simulink model "cic_dezim4_"  (Simulink 7.8)
settings: Solver=FixedStepDiscrete  StartTime=0.0  StopTime=1  RelTol=1e-3
undefined symbols (not defined in the file or in its folder): dfilt
libraries: dspsigops x8, dspsrcs4 x1, dsparch4 x1
settings Model: Creator=svenhoffmann  LastModifiedBy=josef  ExtModeAutoUpdateStatusClock=off
settings OptimizationCC: InlineInvariantSignals=on  InitFltsAndDblsToZero=on
settings DebuggingCC: SaveWithParameterizedLinksMsg=none  SignalResolutionControl=TryResolveAllWithWarning  MultiTaskDSMMsg=warning  MultiTaskCondExecSysMsg=none  FcnCallInpInsideContextMsg=Use local settings  StrictBusMsg=None
settings RTWCC: IncludeERTFirstTime=on
settings GRTTargetCC: TargetFcnLib=ansi_tfl_tmw.mat

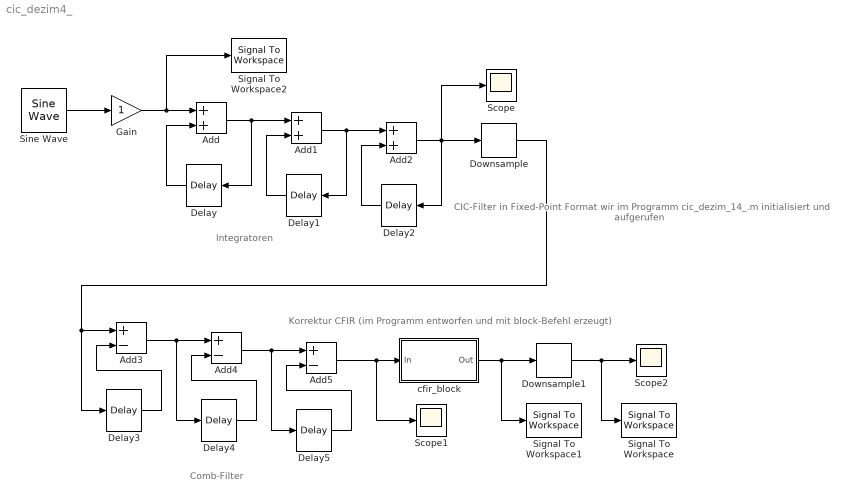
== system cic_dezim4_ ==
  note: Korrektur CFIR (im Programm entworfen
      | und mit block-Befehl erzeugt)
  note: CIC-Filter
      | in Fixed-Point
      | Format
      | wir im Programm
      | cic_dezim_14_.m
      | initialisiert
      | und aufgerufen
  note: Integratoren
  note: Comb-Filter
  Add : Sum  OutDataTypeStr=Inherit: Inherit via back propagation
  Add1 : Sum  OutDataTypeStr=Inherit: Inherit via back propagation
  Add2 : Sum  OutDataTypeStr=Inherit: Inherit via back propagation
  Add3 : Sum  Inputs=+-
  Add4 : Sum  Inputs=+-
  Add5 : Sum  Inputs=+-
  Delay{,1..5} (6 alike) : dspsigops/Delay  InputProcessing=Inherited (this choice will be removed - see release notes)  dly_unit=Samples  delay=1  ic_detail=off  dif_ic_for_ch=off  dif_ic_for_dly=off  ic=0  reset_popup=None
  Downsample : dspsigops/Downsample  N=5  phase=0  InputProcessing=Inherited (this choice will be removed - see release notes)  RateOptions=Enforce single-rate processing  smode=Allow multirate  fmode=Maintain input frame size  ic=0
  Downsample1 : dspsigops/Downsample  N=2  phase=0  InputProcessing=Inherited (this choice will be removed - see release notes)  RateOptions=Enforce single-rate processing  smode=Allow multirate  fmode=Maintain input frame size  ic=0
  Gain : Gain  OutDataTypeStr=fixdt(1,32,10)
  Scope : Scope
  Scope1 : Scope
      settings: YMin=-100  YMax=100
  Scope2 : Scope
      settings: YMin=-100  YMax=100  SaveName=ScopeData2
  Signal To Workspace : SignalToWorkspace  VariableName=yout  SaveFormat=Array
      settings: CopyFcn=dspblkcopystw(gcbh);
  Signal To Workspace1 : SignalToWorkspace  VariableName=yout1  SaveFormat=Array
      settings: CopyFcn=dspblkcopystw(gcbh);
  Signal To Workspace2 : SignalToWorkspace  VariableName=yout2  SaveFormat=Array
      settings: CopyFcn=dspblkcopystw(gcbh);  Decimation=10
  Sine Wave : dspsrcs4/Sine Wave  Amplitude=0.75  Frequency=10000/(fix(10000/50))  Phase=0  SampleMode=Discrete  OutComplex=Real  CompMethod=Table lookup  TableSize=Speed  SampleTime=1/10000  SamplesPerFrame=1  ResetState=Restart at time zero  dataType=Fixed-point  wordLen=16  udDataType=sfix(16)  fracBitsMode=User-defined  numFracBits=15  OutDataTypeStr=fixdt(1,16,15)  LastOutDataTypeStr=fixdt(1,16,15)
  cfir_block : Subsystem  Tag=BlockMethodSubSystem
  wires:
  Sine Wave/1 -> Gain/1
  Delay/1 -> Add/2
  Add/1 -> Delay/1, Add1/1
  Delay1/1 -> Add1/2
  Add1/1 -> Delay1/1, Add2/1
  Add2/1 -> Delay2/1, Scope/1, Downsample/1
  Delay2/1 -> Add2/2
  Delay3/1 -> Add3/2
  Delay4/1 -> Add4/2
  Delay5/1 -> Add5/2
  Add3/1 -> Add4/1, Delay4/1
  Add4/1 -> Add5/1, Delay5/1
  Downsample/1 -> Add3/1, Delay3/1
  Add5/1 -> cfir_block/1(In), Scope1/1
  cfir_block/1(Out) -> Downsample1/1, Signal To Workspace1/1
  Downsample1/1 -> Scope2/1, Signal To Workspace/1
  Gain/1 -> Add/1, Signal To Workspace2/1

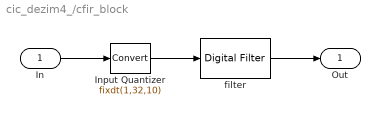
== system cic_dezim4_/cfir_block ==
  In : Inport
  Input Quantizer : DataTypeConversion  OutDataTypeStr=fixdt(1,32,10)  RndMeth=Round  SaturateOnIntegerOverflow=on
  filter : dsparch4/Digital Filter  TypePopup=FIR (all zeros)  IIRFiltStruct=Direct form II transposed  AllPoleFiltStruct=Direct form  FIRFiltStruct=Direct form  CoeffSource=Specify via dialog  NumCoeffs=[0.000150175572468947 0.000679339549982413 0.00146620704190252 0.00176263838807132 0.000358947389225614 -0.00374234854253421 -0.0102890577347766 -0.0168866914876468 -0.0189532635299849 -0.0109674989875637 0.0111898477284377 0.0477264332513376 0.0935414929191431 0.138920854230274 0.172392134336882 0.184725929749563 0.172392134336882 0.138920854230274 0.0935414929191431 0.0477264332513376 0.0111898477284377 -0.0109674989875637 -0.0189532635299849 -0.0168866914876468 -0.0102890577347766 -0.00374234854253421 0.000358947389225614 0.00176263838807132 0.00146620704190252 0.000679339549982413 0.000150175572468947]  DenCoeffs=[1 0.1]  BiQuadCoeffs=[1 0.3 0.4 1 0.1 0.2]  LatticeCoeffs=[0.2 0.4]  denIgnore=on  FiltPerSampPopup=One filter per frame  IC=0  ICnum=0  ICden=0  firstCoeffMode=Binary point scaling  firstCoeffWordLength=16  firstCoeffFracLength=15  outputMode=Binary point scaling  outputWordLength=32  outputFracLength=10  accumMode=Binary point scaling  accumWordLength=64  accumFracLength=32  prodOutputMode=Binary point scaling  prodOutputWordLength=64  prodOutputFracLength=32  roundingMode=Floor  overflowMode=on  ScaleValues=1  scaleValueFracLength=14  stageInFracLength=15  stageOutFracLength=15  FilterSource=Specify via dialog  dfiltObjectName=dfilt.dffir([1 2 1])  InputProcessing=Columns as channels (frame based)
  Out : Outport
  wires:
  In/1 -> Input Quantizer/1
  Input Quantizer/1 -> filter/1
  filter/1 -> Out/1
